simulink model "Sim_Induct"  (R2019a)
settings: Solver=FixedStepAuto  StartTime=0.0  StopTime=sim_time  FixedStep=1e-6  MaxStep=1e-4  RelTol=1e-3
values from neighbouring files (symbols this model uses):
  C21 = 100e-6    (= 0.0001)    [main_simu.m]
  C22 = 100e-6    (= 0.0001)    [main_simu.m]
  C23 = 220e-6    (= 0.00022)    [main_simu.m]
  C24 = 330e-6    (= 0.00033)    [main_simu.m]
  L41 = 10e-3    (= 0.01)    [main_simu.m]
  L42 = 10e-3    (= 0.01)    [main_simu.m]
  L43 = 10e-3    (= 0.01)    [main_simu.m]
  L44 = 100e-3    (= 0.1)    [main_simu.m]
  L61 = 1e-3    (= 0.001)    [main_simu.m]
  L62 = 1e-3    (= 0.001)    [main_simu.m]
  L63 = 1e-3    (= 0.001)    [main_simu.m]
  L64 = 1e-3    (= 0.001)    [main_simu.m]
  R21 = 2e3    (= 2000)    [main_simu.m]
  R22 = 1e3    (= 1000)    [main_simu.m]
  R23 = 500    [main_simu.m]
  R24 = 300    [main_simu.m]
  R31 = 2.5    [main_simu.m]
  R32 = 5    [main_simu.m]
  R33 = 8    [main_simu.m]
  R34 = 10    [main_simu.m]
  R41 = 10    [main_simu.m]
  R42 = 20    [main_simu.m]
  R43 = 30    [main_simu.m]
  R44 = 30    [main_simu.m]
  R51 = 10    [main_simu.m]
  R52 = 12    [main_simu.m]
  R53 = 15    [main_simu.m]
  R54 = 20    [main_simu.m]
  R61 = 10    [main_simu.m]
  R62 = 5    [main_simu.m]
  R63 = 30    [main_simu.m]
  R64 = 105    [main_simu.m]
  R71 = 5    [main_simu.m]
  R72 = 10    [main_simu.m]
  R73 = 20    [main_simu.m]
  R74 = 50    [main_simu.m]
  sim_off = sim_on    [main_simu.m]    (also in quintuple_load.m; sevenfold_load.m; sixfold_load.m)
  sim_on = 50*ones(1,num_loads)    [main_simu.m]    (also in quintuple_load.m = 50*ones(1,28); sevenfold_load.m = 50*ones(1,28); sixfold_load.m = 50*ones(1,28))
  Valpha5 = 60    [main_simu.m]
  Valpha6 = 60    [main_simu.m]
undefined symbols (not defined in the file or in its folder): J, Laq, Lse, R, Ra, Rse, SEIP4, SEVP4, wm0, wmo
libraries: powerlib x206, simulink x72
(part 3 of 3)

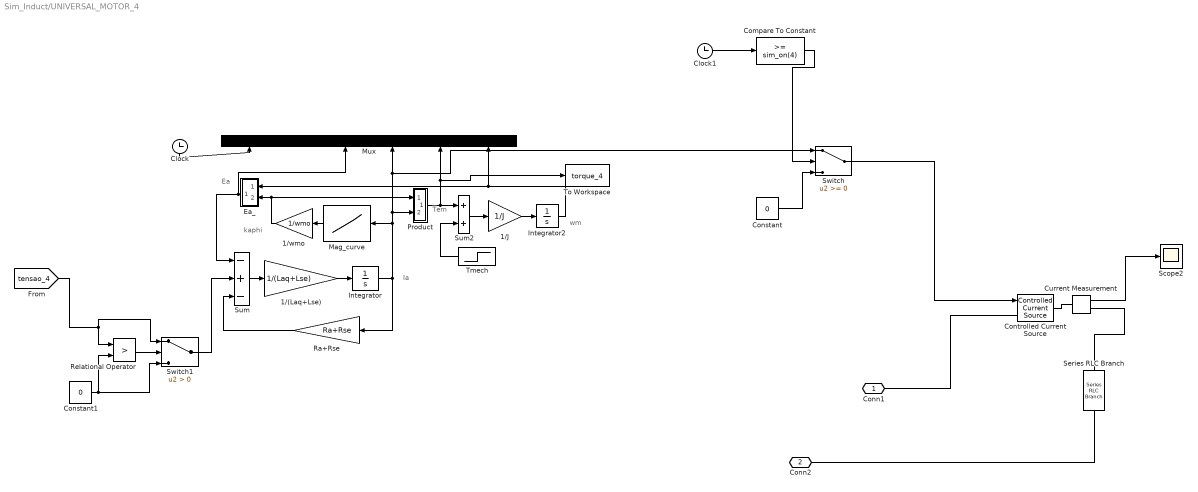
== system Sim_Induct/UNIVERSAL_MOTOR_4 ==
  note: kaphi
  note: Tem
  note: Ea
  note: wm
  note: Ia
  1/(Laq+Lse) : Gain  Gain=1/(Laq+Lse)  SaturateOnIntegerOverflow=on  OutDataTypeStr=Inherit: Same as input  ParamDataTypeStr=Inherit: Same as input
  1/J : Gain  Gain=1/J  SaturateOnIntegerOverflow=on  OutDataTypeStr=Inherit: Same as input  ParamDataTypeStr=Inherit: Same as input
  1/wmo : Gain  Gain=1/wmo  SaturateOnIntegerOverflow=on  OutDataTypeStr=Inherit: Same as input  ParamDataTypeStr=Inherit: Same as input
  Clock : Clock
  Clock1 : Clock
  Compare To Constant : simulink/Logic and Bit Operations/Compare To Constant  relop=>=  const=sim_on(4)  OutDataTypeStr=boolean
  Constant : Constant  Value=0
  Constant1 : Constant  Value=0
  Controlled Current Source : powerlib/Electrical Sources/Controlled Current Source  Initialize=on  Source_Type=AC  Amplitude=0  Phase=0  Frequency=0  Measurements=None
      settings: SourceProductName=Simscape Electrical
  Current Measurement : powerlib/Measurements/Current Measurement  PhasorSimulation=off  OutputType=Complex  PSBequivalent=0
      settings: SourceProductName=Simscape Electrical
  Ea_ : Subsystem  mask(Dot Product){}
      mask help:
      | Inner (dot) product.
      | y=sum(u1.*u2)
      mask Help: Computes the inner (dot) product of the inputs: sum(u1.*u2).  The inputs are vectors of the same length. Output is a scalar.
      mask Display: disp('.\n')
  Integrator : Integrator
  Integrator2 : Integrator  InitialCondition=wm0
  Mag_curve : Lookup  InputValues=SEIP4  Table=SEVP4  SaturateOnIntegerOverflow=on
  Mux : Mux  Inputs=6
  Product : Subsystem  mask(Dot Product){}
      mask help:
      | Inner (dot) product.
      | y=sum(u1.*u2)
      mask Help: Computes the inner (dot) product of the inputs: sum(u1.*u2).  The inputs are vectors of the same length. Output is a scalar.
      mask Display: disp('.\n')
  Ra+Rse : Gain  Gain=Ra+Rse  SaturateOnIntegerOverflow=on  OutDataTypeStr=Inherit: Same as input  ParamDataTypeStr=Inherit: Same as input
  Relational Operator : RelationalOperator  Operator=>  OutDataTypeStr=boolean  RndMeth=Simplest
  Scope2 : Scope
  Series RLC Branch : powerlib/Elements/Series RLC Branch  LConnTagsString=__new0  RConnTagsString=__new0  BranchType=R  Resistance=1e-15  Inductance=1e-3  SetiL0=off  InitialCurrent=0  Capacitance=1e-6  Setx0=off  InitialVoltage=0  Measurements=None
      settings: SourceProductName=Simscape Electrical
  Sum : Sum  Inputs=-+-  SaturateOnIntegerOverflow=on  InputSameDT=on  OutDataTypeStr=Inherit: Same as first input
  Sum2 : Sum  SaturateOnIntegerOverflow=on  InputSameDT=on  OutDataTypeStr=Inherit: Same as first input
  Switch : Switch
  Switch1 : Switch  Criteria=u2 > Threshold
  Tmech : Step  Time=0  Before=-0.8  After=0.5
  To Workspace : ToWorkspace  VariableName=torque_4  SaveFormat=Timeseries  SampleTime=-1
  Conn1 : PMIOPort  Side=Left
  Conn2 : PMIOPort  Port=2  Side=Left
  wires:
  Ra+Rse/1 -> Sum/3
  1/J/1 -> Integrator2/1
  1/wmo/1 -> Ea_/2(in_2), Product/1(in_1)
  Current Measurement/1 -> Scope2/1
  Mag_curve/1 -> 1/wmo/1
  Sum/1 -> 1/(Laq+Lse)/1
  Sum2/1 -> 1/J/1
  1/(Laq+Lse)/1 -> Integrator/1
  Ea_/1(out_1) -> Mux/3, Sum/1
  Integrator2/1 -> Mux/6, Ea_/1(in_1)
  Tmech/1 -> Sum2/2
  Integrator/1 -> Switch/1, Mux/4, Product/2(in_2), Mag_curve/1, Ra+Rse/1
  Clock/1 -> Mux/1
  Product/1(out_1) -> To Workspace/1, Mux/5, Sum2/1
  Constant/1 -> Switch/3
  Compare To Constant/1 -> Switch/2
  Clock1/1 -> Compare To Constant/1
  Switch/1 -> Controlled Current Source/1
  Relational Operator/1 -> Switch1/2
  Constant1/1 -> Relational Operator/2, Switch1/3
  Switch1/1 -> Sum/2
  [tensao_4] -> Relational Operator/1, Switch1/1
  connections:
  Conn2/RConn1 -- Series RLC Branch/RConn1
  Controlled Current Source/LConn1 -- Conn1/RConn1
  Current Measurement/LConn1 -- Controlled Current Source/RConn1
  Current Measurement/RConn1 -- Series RLC Branch/LConn1

== system Sim_Induct/UNIVERSAL_MOTOR_1/Ea_ ==
  in_1 : Inport
  in_2 : Inport  Port=2
  Product : Product  SaturateOnIntegerOverflow=on  RndMeth=Zero  InputSameDT=on  OutDataTypeStr=Inherit: Same as first input
  Sum : Sum  Inputs=+  SaturateOnIntegerOverflow=on  InputSameDT=on  OutDataTypeStr=Inherit: Same as first input
  out_1 : Outport  InitialOutput=0
  wires:
  Sum/1 -> out_1/1
  Product/1 -> Sum/1
  in_1/1 -> Product/1
  in_2/1 -> Product/2

== system Sim_Induct/UNIVERSAL_MOTOR_1/Product ==
  in_1 : Inport
  in_2 : Inport  Port=2
  Product : Product  SaturateOnIntegerOverflow=on  RndMeth=Zero  InputSameDT=on  OutDataTypeStr=Inherit: Same as first input
  Sum : Sum  Inputs=+  SaturateOnIntegerOverflow=on  InputSameDT=on  OutDataTypeStr=Inherit: Same as first input
  out_1 : Outport  InitialOutput=0
  wires:
  Sum/1 -> out_1/1
  Product/1 -> Sum/1
  in_1/1 -> Product/1
  in_2/1 -> Product/2

== system Sim_Induct/UNIVERSAL_MOTOR_2/Ea_ ==
  in_1 : Inport
  in_2 : Inport  Port=2
  Product : Product  SaturateOnIntegerOverflow=on  RndMeth=Zero  InputSameDT=on  OutDataTypeStr=Inherit: Same as first input
  Sum : Sum  Inputs=+  SaturateOnIntegerOverflow=on  InputSameDT=on  OutDataTypeStr=Inherit: Same as first input
  out_1 : Outport  InitialOutput=0
  wires:
  Sum/1 -> out_1/1
  Product/1 -> Sum/1
  in_1/1 -> Product/1
  in_2/1 -> Product/2

== system Sim_Induct/UNIVERSAL_MOTOR_2/Product ==
  in_1 : Inport
  in_2 : Inport  Port=2
  Product : Product  SaturateOnIntegerOverflow=on  RndMeth=Zero  InputSameDT=on  OutDataTypeStr=Inherit: Same as first input
  Sum : Sum  Inputs=+  SaturateOnIntegerOverflow=on  InputSameDT=on  OutDataTypeStr=Inherit: Same as first input
  out_1 : Outport  InitialOutput=0
  wires:
  Sum/1 -> out_1/1
  Product/1 -> Sum/1
  in_1/1 -> Product/1
  in_2/1 -> Product/2

== system Sim_Induct/UNIVERSAL_MOTOR_3/Ea_ ==
  in_1 : Inport
  in_2 : Inport  Port=2
  Product : Product  SaturateOnIntegerOverflow=on  RndMeth=Zero  InputSameDT=on  OutDataTypeStr=Inherit: Same as first input
  Sum : Sum  Inputs=+  SaturateOnIntegerOverflow=on  InputSameDT=on  OutDataTypeStr=Inherit: Same as first input
  out_1 : Outport  InitialOutput=0
  wires:
  Sum/1 -> out_1/1
  Product/1 -> Sum/1
  in_1/1 -> Product/1
  in_2/1 -> Product/2

== system Sim_Induct/UNIVERSAL_MOTOR_3/Product ==
  in_1 : Inport
  in_2 : Inport  Port=2
  Product : Product  SaturateOnIntegerOverflow=on  RndMeth=Zero  InputSameDT=on  OutDataTypeStr=Inherit: Same as first input
  Sum : Sum  Inputs=+  SaturateOnIntegerOverflow=on  InputSameDT=on  OutDataTypeStr=Inherit: Same as first input
  out_1 : Outport  InitialOutput=0
  wires:
  Sum/1 -> out_1/1
  Product/1 -> Sum/1
  in_1/1 -> Product/1
  in_2/1 -> Product/2

== system Sim_Induct/UNIVERSAL_MOTOR_4/Ea_ ==
  in_1 : Inport
  in_2 : Inport  Port=2
  Product : Product  SaturateOnIntegerOverflow=on  RndMeth=Zero  InputSameDT=on  OutDataTypeStr=Inherit: Same as first input
  Sum : Sum  Inputs=+  SaturateOnIntegerOverflow=on  InputSameDT=on  OutDataTypeStr=Inherit: Same as first input
  out_1 : Outport  InitialOutput=0
  wires:
  Sum/1 -> out_1/1
  Product/1 -> Sum/1
  in_1/1 -> Product/1
  in_2/1 -> Product/2

== system Sim_Induct/UNIVERSAL_MOTOR_4/Product ==
  in_1 : Inport
  in_2 : Inport  Port=2
  Product : Product  SaturateOnIntegerOverflow=on  RndMeth=Zero  InputSameDT=on  OutDataTypeStr=Inherit: Same as first input
  Sum : Sum  Inputs=+  SaturateOnIntegerOverflow=on  InputSameDT=on  OutDataTypeStr=Inherit: Same as first input
  out_1 : Outport  InitialOutput=0
  wires:
  Sum/1 -> out_1/1
  Product/1 -> Sum/1
  in_1/1 -> Product/1
  in_2/1 -> Product/2
